simulink model "minimalist08_noMPC_01"  (Simulink 7.4)
settings: Solver=FixedStepDiscrete  StartTime=0.0  StopTime=inf  RelTol=1e-3
PreLoadFcn:
  | RTWConfigurationCB('preloadfcn', bdroot);
PostLoadFcn:
  | mpc555rt_switch_target(gcs,'auto')
CloseFcn:
  | rtwprivate ssgencode ModelCloseRequest foo
settings Model: Creator=The MathWorks Inc.  LastModifiedBy=autopilot
settings DataIOCC: LimitDataPoints=off  SignalLoggingName=sigsOut
settings OptimizationCC: InlineParams=on  InlineInvariantSignals=on  EnforceIntegerDowncast=off  ZeroExternalMemoryAtStartup=off  ZeroInternalMemoryAtStartup=off  InitFltsAndDblsToZero=on  NoFixptDivByZeroProtection=on  OptimizeModelRefInitCode=on  LifeSpan=1
settings DebuggingCC: SaveWithParameterizedLinksMsg=none  SignalResolutionControl=TryResolveAllWithWarning  SolverPrmCheckMsg=none  MultiTaskDSMMsg=warning  MultiTaskCondExecSysMsg=none  UnderSpecifiedDataTypeMsg=error  StrictBusMsg=None
settings HardwareCC: ProdEndianess=BigEndian  ProdHWDeviceType=Motorola PowerPC
settings RTWCC: SystemTargetFile=mpc555rt.tlc  TemplateMakefile=mpc555rt.tmf  Description=Target Support Package (for use with Freescale MPC5xx) (real-time)  ProcessScript=mpc555rt_make_rtw_hook
settings CodeAppCC: IgnoreCustomStorageClasses=off
settings STFCustomTargetCC: TargetFcnLib=ansi_tfl_tmw.mat  TargetLibSuffix=.a  TargetPreCompLibLocation=C:\Program Files\MATLAB\R2009b\toolbox\rtw\targets\mpc555dk\drivers\lib\DIAB  IncludeMdlTerminateFcn=off  CombineOutputUpdateFcns=on  ERTCustomFileBanners=on  SupportAbsoluteTime=off  SupportNonFinite=off  SupportComplex=off  SupportContinuousTime=off  SupportNonInlinedSFcns=off  CPPClassGenCompliant=on  SystemTargetFile=mpc555rt.tlc
settings ERTTargetCC: TargetFcnLib=ansi_tfl_tmw.mat  TargetPreCompLibLocation=C:\Program Files\MATLAB\R2009b\toolbox\rtw\targets\mpc555dk\drivers\lib\DIAB  MultiwordLength=2048  ParMdlRefBuildCompliant=off  CompOptLevelCompliant=off  IncludeMdlTerminateFcn=off  ERTFirstTimeCompliant=off  SupportAbsoluteTime=off  SupportNonFinite=off  SupportComplex=off  ModelStepFunctionPrototypeControlCompliant=off  ExtModeMexFile=MPC5xxExternalModeOpen  ExtModeIntrfLevel=Level2 - Open  ERTCustomFileTemplate=example_file_process.tlc  ConvertIfToSwitch=off
settings CustomProperty: DataType=RTWOptions_EnumType__toolbox_rtw_targets_mpc555dk_mpc555dk_mpc555rt_1MPC555_OPTIMIZATION_SWITCH  Value=speed
settings EnumStrPairs: String=speed

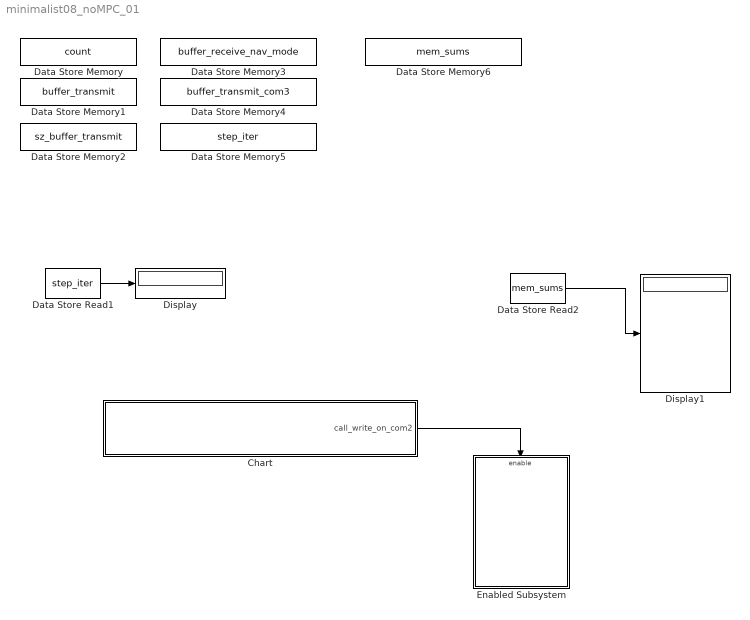
== system minimalist08_noMPC_01 ==
  Chart : Stateflow chart
  Data Store Memory : DataStoreMemory  DataStoreName=count  DataType=uint8  OutDataType=fixdt(1, 16)  OutScaling=2^0  OutDataTypeStr=uint8
  Data Store Memory1 : DataStoreMemory  DataStoreName=buffer_transmit  InitialValue=[0 0 0 0 0 0 0 0 0 0 0]  DataType=uint8  OutDataType=fixdt(1, 16)  OutScaling=2^0  OutDataTypeStr=uint8
  Data Store Memory2 : DataStoreMemory  DataStoreName=sz_buffer_transmit  DataType=uint32  OutDataType=fixdt(1, 16)  OutScaling=2^0  OutDataTypeStr=uint32
  Data Store Memory3 : DataStoreMemory  DataStoreName=buffer_receive_nav_mode  InitialValue=[0 0 0 0 0 0 0 0 0 0 0 0 0 0 0 0 0 0 0 0 0 0 0 0 0 0 0 0 0 0 0 0 0 0 0 0 0]  DataType=uint8  OutDataType=fixdt(1, 16)  OutScaling=2^0  OutDataTypeStr=uint8
  Data Store Memory4 : DataStoreMemory  DataStoreName=buffer_transmit_com3  InitialValue=[1]  DataType=uint8  OutDataType=fixdt(1, 16)  OutScaling=2^0  OutDataTypeStr=uint8
  Data Store Memory5 : DataStoreMemory  DataStoreName=step_iter  DataType=uint8  OutDataType=fixdt(1, 16)  OutScaling=2^0  OutDataTypeStr=uint8
  Data Store Memory6 : DataStoreMemory  DataStoreName=mem_sums  InitialValue=[0 0 0]  DataType=uint32  OutDataType=fixdt(1, 16)  OutScaling=2^0  OutDataTypeStr=uint32
  Data Store Read1 : DataStoreRead  DataStoreName=step_iter  SampleTime=-1
  Data Store Read2 : DataStoreRead  DataStoreName=mem_sums  SampleTime=-1
  Display : Display
  Display1 : Display
  Enabled Subsystem : Subsystem  TreatAsAtomicUnit=on
  wires:
  Chart/1(call_write_on_com2) -> Enabled Subsystem/Enable
  Data Store Read1/1 -> Display/1
  Data Store Read2/1 -> Display1/1

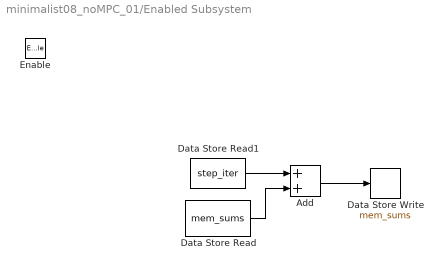
== system minimalist08_noMPC_01/Enabled Subsystem ==
  Enable : EnablePort
  Add : Sum  AccumDataTypeStr=uint32  OutDataTypeMode=uint32  OutDataType=fixdt(1, 16)  OutScaling=2^-10  OutDataTypeStr=uint32
  Data Store Read : DataStoreRead  DataStoreName=mem_sums  SampleTime=0
  Data Store Read1 : DataStoreRead  DataStoreName=step_iter  SampleTime=-1
  Data Store Write : DataStoreWrite  DataStoreName=mem_sums  SampleTime=-1
  wires:
  Data Store Read1/1 -> Add/1
  Data Store Read/1 -> Add/2
  Add/1 -> Data Store Write/1

== stateflow chart Chart ==
  state STEP01
    call_write_on_com2=1;
    step_iter = step_iter + 1;
  state STEP02
    call_write_on_com2=0;
  STEP01 -> STEP02 [order 2] : [step_iter>=250]
  STEP01 -> STEP01 [order 1] : [step_iter<250]
  (default) -> STEP01
  data: step_iter data_store_memory double; call_write_on_com2 output uint8
